simulink model "Z_3DCtrl_xiaodong"  (R2022a)
settings: Solver=ode1  StartTime=0.0  StopTime=Inf  FixedStep=0.001  RelTol=1e-3  EnableMultiTasking=on
PostLoadFcn:
  | , if any(exist('dsrtsu_mdlpostloadfcn', 'file') ~= 0), dsrtsu_mdlpostloadfcn('Execute', bdroot); end,
InitFcn:
  | , if any(exist('rtifpga_mdlclblib', 'file') ~= 0), rtifpga_mdlclblib('Init', bdroot); end,
  | [b,a] = butter(6,0.6)
undefined symbols (not defined in the file): a, b, DiscIntNeverNeededParam
libraries: simulink x3, rti2004lib x3, rtilibm x1
settings Model: DSRTSU_INTERNAL_RTI_VER=600  DSRTSU_INTERNAL_RTI_TYPE=rti1006  DSRTSU_INTERNAL_RTIFPGA=180  DSRTSU_INTERNAL_RTISTBM_VER=1.4.4  Creator=Administrator  LastModifiedBy=jnofech
settings SolverCC: AlgebraicLoopSolver=TrustRegion
settings DataIOCC: LimitDataPoints=on  SaveFormat=Array  SignalLoggingSaveFormat=ModelDataLogs  ReturnWorkspaceOutputs=off
settings OptimizationCC: BlockReduction=off  OptimizeBlockIOStorage=off  BufferReuse=off  ExpressionFolding=off  ExpressionDepthLimit=2147483647  LocalBlockOutputs=off  LifeSpan=inf
settings DebuggingCC: UnderspecifiedInitializationDetection=Classic  MergeDetectMultiDrivingBlocksExec=none  SolverPrmCheckMsg=warning  FcnCallInpInsideContextMsg=warning  UnconnectedInputMsg=warning  UnconnectedOutputMsg=warning  UnconnectedLineMsg=warning  StateNameClashWarn=warning  SFUnexpectedBacktrackingDiag=warning  SFNoUnconditionalDefaultTransitionDiag=warning  SFExecutionAtInitializationDiag=none  SFMachineParentedDataDiag=warning  ArithmeticOperatorsInVariantConditions=warning
settings HardwareCC: ProdBitPerPointer=32  ProdBitPerSizeT=32  ProdBitPerPtrDiffT=32  ProdLargestAtomicInteger=Integer  ProdWordSize=32  ProdHWDeviceType=Custom Processor->Custom  TargetIntDivRoundTo=Zero  TargetEndianess=LittleEndian  TargetHWDeviceType=Custom Processor->Custom
settings ModelReferenceCC: PropagateSignalLabelsOutOfModel=off
settings SFSimCC: SimUseLocalCustomCode=off  MATLABDynamicMemAlloc=off  CustomCodeUndefinedFunction=UseInterfaceOnly
settings RTWCC: Description=dSPACE DS1006 Hardware Platform  SystemTargetFile=rti1006.tlc  MakeCommand=make_rti  TemplateMakefile=rti1006.tmf  RTWUseLocalCustomCode=off
settings CodeAppCC: StateflowObjectComments=on
settings STFCustomTargetCC: ParMdlRefBuildCompliant=on  GRTInterface=off  SystemTargetFile=rti1006.tlc
settings GRTTargetCC: TargetLangStandard=C89/C90 (ANSI)  CompOptLevelCompliant=off  ConcurrentExecutionCompliant=off  CombineOutputUpdateFcns=off  MatFileLogging=off  CPPClassGenCompliant=off  UseToolchainInfoCompliant=off  ExtModeMexFile=noextcomm
settings ConfigComp: CovMetricSettings=dw  CovSaveCumulativeToWorkspaceVar=on  CovSaveSingleToWorkspaceVar=on

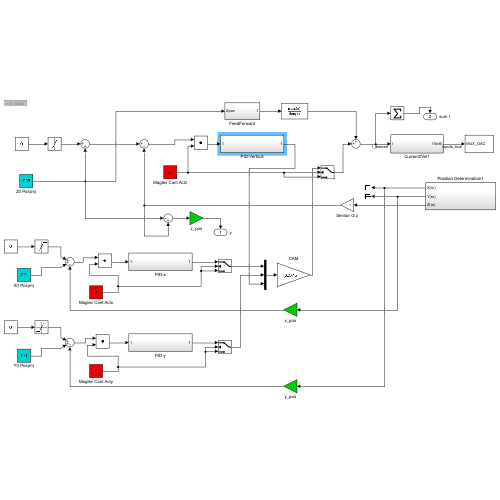
[thumbnail: Simulink's stored preview of the top-level diagram]
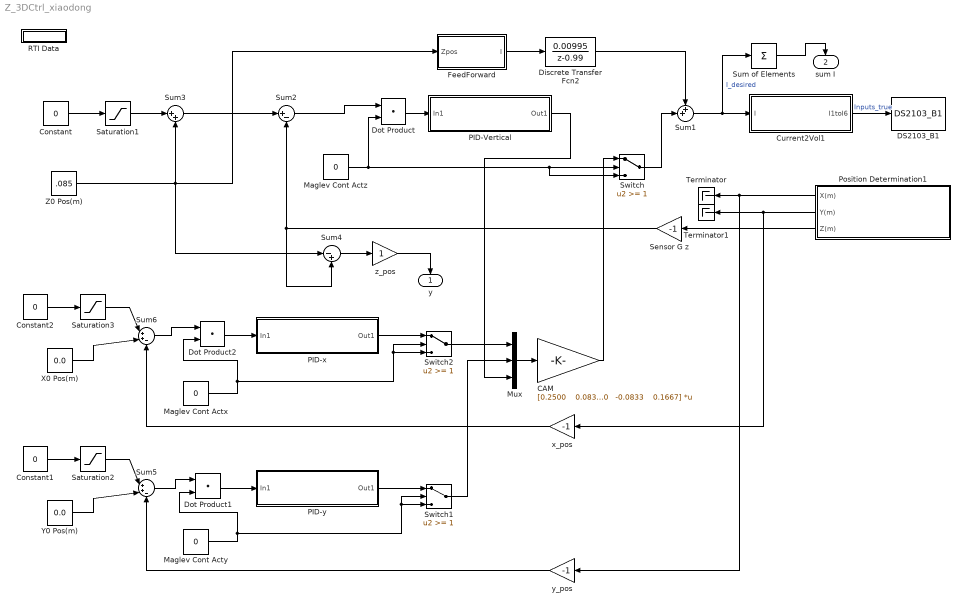
== system Z_3DCtrl_xiaodong ==
  CAM : Gain  Gain=|  Multiplication=Matrix(K*u)
      | [0.2500    0.0833    0.1667
      |          0    0.1667    0.1667
      |    -0.2500    0.0833    0.1667
      |    -0.2500   -0.0833    0.1667
      |          0   -0.1667    0.1667
      |     0.2500   -0.0833    0.1667]
  Constant : Constant  Value=0
  Constant1 : Constant  Value=0
  Constant2 : Constant  Value=0
  Current2Vol1 : Subsystem
  DS2103_B1 : rtilibm/DS2103/DS2103_B1  BoardNo=1  ChannelNos=[1 2 4 6 8 9 10 11 12 18 19 20]  Range=[10 10 10 10 10 10 10 10 10 10 10 10 10 10 10 10 10 10 10 10 10 10 10 10 10 10 10 10 10 10 10 10]  IOErrorMode=[1 1 1 1 1 1 1 1]  InitValue=[0 0 0 0 0 0 0 0 0 0 0 0 0 0 0 0 0 0 0 0 0 0 0 0 0 0 0 0 0 0 0 0]  TermMode=[0 0 0 0 0 0 0 1 1 1 1 1 1 1 1 1 1 1 1 1 1 1 1 1 1 1 1 1 1 1 1 1]  TermValue=[0 0 0 0 0 0 0 0 0 0 0 0 0 0 0 0 0 0 0 0 0 0 0 0 0 0 0 0 0 0 0 0]  DialogFcn=gui2103  UnitName={ 'DS2103_B' }  UnitValues={ 1 }  DSProperties=struct('RTI',struct('Version',uint32(1),'BlockType',struct('isSLSource',uint8(0),'isSLSink',uint8(1),'isHWSource',uint8(0),'isHWSink',uint8(1),'isSetup',uint8(0),'isInline',uint8(1),'isNonInline',uint8(0),'isInterrupt',uint8(0),'isChannelwise',uint8(0)),'IOBoardType','DS2103','UnitType','DAC','Identifier','DACMUX','DialogType','ML','BlockSet','NONE','SlaveProcessor','NONE'))
      settings: SourceProductName=dSPACE RTI1006
  Discrete Transfer Fcn2 : DiscreteTransferFcn  Numerator=[0.00995]  Denominator=[1 -0.99]
  Dot Product : DotProduct  OutDataTypeStr=Inherit: Inherit via internal rule
  Dot Product1 : DotProduct  OutDataTypeStr=Inherit: Inherit via internal rule
  Dot Product2 : DotProduct  OutDataTypeStr=Inherit: Inherit via internal rule
  FeedForward : Subsystem
  Maglev Cont Actx : Constant  Value=0
  Maglev Cont Acty : Constant  Value=0
  Maglev Cont Actz : Constant  Value=0
  Mux : Mux  Inputs=3
  PID-Vertical : Subsystem
  PID-x : Subsystem
  PID-y : Subsystem
  Position Determination1 : Subsystem
  RTI Data : Subsystem  Tag=struct('RTIDataServer',struct('RTIDataServerVs','2','RTIModelDescription','struct(''main'',''Z_3DCtrl_xiaodong'',''sub'','''',''isMp'',0)'))  LoadFcn="if exist('rtidc'), try,  rtidc('DataHostBlockClbLoad', gcbh); catch, disp(['Warning: ''LoadFcn'' for RTI Data block failed: ' lasterr]); end, end,"  mask(RTI_DATA_HOST){}
      mask help:
      | RTI Data Block.
      | This block is used by RTI to store internal model-dependent data.
      | Please keep this block on the root level of the model. Deleting this block will result in data loss.
      |
      | NEVER DELETE OR COPY THIS BLOCK!
      settings: CopyFcn="if exist('rtidc'), try,  rtidc('DataHostBlockClbCopy', gcbh); catch, disp(['Warning: ''CopyFcn'' for RTI Data block failed: ' lasterr]); end, end,"  DeleteFcn="if exist('rtidc'), try,  rtidc('DataHostBlockClbDelete', gcbh); catch, disp(['Warning: ''DeleteFcn'' for RTI Data block failed: ' lasterr]); end, end,"  ModelCloseFcn="if exist('rtidc'), try,  rtidc('DataHostBlockClbModelClose', gcbh); catch, disp(['Warning: ''ModelCloseFcn'' for RTI Data block failed: ' lasterr]); end, end,"  PreSaveFcn="if exist('rtidc'), try,  rtidc('DataHostBlockClbPreSave', gcbh); catch, disp(['Warning: ''PreSaveFcn'' for RTI Data block failed: ' lasterr]); end, end,"  PostSaveFcn="if exist('rtidc'), try,  rtidc('DataHostBlockClbPostSave', gcbh); catch, disp(['Warning: ''PostSaveFcn'' for RTI Data block failed: ' lasterr]); end, end,"  NameChangeFcn="if exist('rtidc'), try,  rtidc('DataHostBlockClbNameChange', gcbh); catch, disp(['Warning: ''NameChangeFcn'' for RTI Data block failed: ' lasterr]); end, end,"
      mask Help:
      | RTI Data Block.
      | This block is used by RTI to store internal model-dependent data.
      | Please keep this block on the root level of the model. Deleting this block will result in data loss.
      | 
      | NEVER DELETE OR COPY THIS BLOCK!
      mask Display:
      | text(0.5, 0.5, 'RTI Data', 'HorizontalAlignment', 'center');
      | plot([1 0]);
  Saturation1 : Saturate  UpperLimit=.015  LowerLimit=-.015
  Saturation2 : Saturate  UpperLimit=.01  LowerLimit=-.01
  Saturation3 : Saturate  UpperLimit=.01  LowerLimit=-.01
  Sensor G z : Gain  Gain=-1
  Sum of Elements : Sum  Inputs=+
  Sum1 : Sum  Inputs=++|
  Sum2 : Sum  Inputs=|+-
  Sum3 : Sum  Inputs=|++
  Sum4 : Sum  Inputs=|-+
  Sum5 : Sum  Inputs=|++-
  Sum6 : Sum  Inputs=|++-
  Switch : Switch  Threshold=1  SaturateOnIntegerOverflow=off  InputSameDT=off
  Switch1 : Switch  Threshold=1  SaturateOnIntegerOverflow=off  InputSameDT=off
  Switch2 : Switch  Threshold=1  SaturateOnIntegerOverflow=off  InputSameDT=off
  Terminator : Terminator
  Terminator1 : Terminator
  X0 Pos(m) : Constant  Value=0.0
  Y0 Pos(m) : Constant  Value=0.0
  Z0 Pos(m) : Constant  Value=.085
  x_pos : Gain  Gain=-1
  y_pos : Gain  Gain=-1
  z_pos : Gain
  y : Outport
  sum I : Outport  Port=2
  wires:
  Sum1/1 -> Sum of Elements/1, Current2Vol1/1(I)  "I_desired"
  Sum3/1 -> Sum2/1
  Position Determination1/3(Z(m)) -> Sensor G z/1
  Position Determination1/1(X(m)) -> Terminator/1, y_pos/1
  Position Determination1/2(Y(m)) -> Terminator1/1, x_pos/1
  Sensor G z/1 -> Sum2/2, Sum4/2
  FeedForward/1(I) -> Discrete Transfer Fcn2/1
  Constant/1 -> Saturation1/1
  Saturation1/1 -> Sum3/1
  Sum4/1 -> z_pos/1
  Maglev Cont Actz/1 -> Switch/2, Switch/3, Dot Product/2
  Switch/1 -> Sum1/2
  Dot Product/1 -> PID-Vertical/1(In1)
  Sum2/1 -> Dot Product/1
  Mux/1 -> CAM/1
  CAM/1 -> Switch/1
  PID-Vertical/1(Out1) -> Mux/3
  Constant1/1 -> Saturation2/1
  Saturation2/1 -> Sum5/1
  Discrete Transfer Fcn2/1 -> Sum1/1
  Sum of Elements/1 -> sum I/1
  Sum5/1 -> Dot Product1/1
  Dot Product1/1 -> PID-y/1(In1)
  Maglev Cont Acty/1 -> Dot Product1/2, Switch1/3, Switch1/2
  PID-y/1(Out1) -> Switch1/1
  Switch1/1 -> Mux/2
  Constant2/1 -> Saturation3/1
  Saturation3/1 -> Sum6/1
  Sum6/1 -> Dot Product2/1
  Dot Product2/1 -> PID-x/1(In1)
  Maglev Cont Actx/1 -> Switch2/2, Switch2/3, Dot Product2/2
  PID-x/1(Out1) -> Switch2/1
  Switch2/1 -> Mux/1
  X0 Pos(m)/1 -> Sum6/2
  Y0 Pos(m)/1 -> Sum5/2
  Z0 Pos(m)/1 -> Sum3/2, FeedForward/1(Zpos), Sum4/1
  x_pos/1 -> Sum6/3
  y_pos/1 -> Sum5/3
  z_pos/1 -> y/1
  Current2Vol1/1(I1toI6) -> DS2103_B1/1  "Inputs_true"

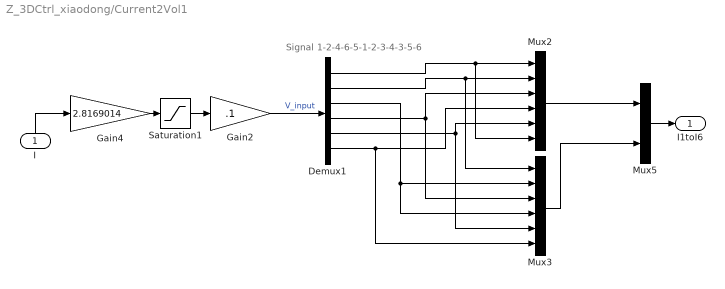
== system Z_3DCtrl_xiaodong/Current2Vol1 ==
  note: Signal 1-2-4-6-5-1-2-3-4-3-5-6
  I : Inport
  Demux1 : Demux  Outputs=6
  Gain2 : Gain  Gain=.1
  Gain4 : Gain  Gain=2.8169014
  Mux2 : Mux  Inputs=6
  Mux3 : Mux  Inputs=6
  Mux5 : Mux  Inputs=2
  Saturation1 : Saturate  UpperLimit=8.2  LowerLimit=0
  I1toI6 : Outport
  wires:
  Mux5/1 -> I1toI6/1
  I/1 -> Gain4/1
  Gain4/1 -> Saturation1/1
  Mux2/1 -> Mux5/1
  Saturation1/1 -> Gain2/1
  Gain2/1 -> Demux1/1  "V_input"
  Mux3/1 -> Mux5/2
  Demux1/1 -> Mux2/1, Mux2/6
  Demux1/2 -> Mux2/2, Mux3/1
  Demux1/4 -> Mux2/3, Mux3/3
  Demux1/6 -> Mux2/4, Mux3/6
  Demux1/5 -> Mux2/5, Mux3/5
  Demux1/3 -> Mux3/2, Mux3/4

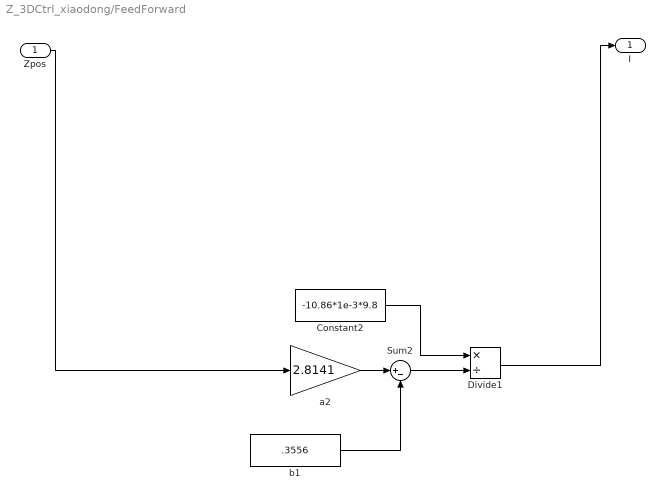
== system Z_3DCtrl_xiaodong/FeedForward ==
  Zpos : Inport
  Constant2 : Constant  Value=-10.86*1e-3*9.8
  Divide1 : Product  Inputs=*/
  Sum2 : Sum  Inputs=|+-
  a2 : Gain  Gain=2.8141
  b1 : Constant  Value=.3556
  I : Outport
  wires:
  a2/1 -> Sum2/1
  b1/1 -> Sum2/2
  Zpos/1 -> a2/1
  Constant2/1 -> Divide1/1
  Sum2/1 -> Divide1/2
  Divide1/1 -> I/1

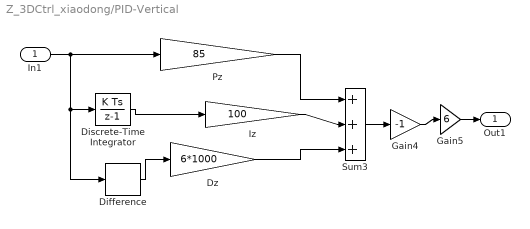
== system Z_3DCtrl_xiaodong/PID-Vertical ==
  In1 : Inport
  Difference : simulink/Discrete/Difference  ICPrevInput=0.0  OutMin=[]  OutMax=[]  OutDataType=sfix(16)  OutScaling=2^-10  DoSatur=off
  Discrete-Time Integrator : DiscreteIntegrator  SampleTime=-1  ICPrevOutput=DiscIntNeverNeededParam  ICPrevScaledInput=DiscIntNeverNeededParam
  Dz : Gain  Gain=6*1000
  Gain4 : Gain  Gain=-1
  Gain5 : Gain  Gain=6
  Iz : Gain  Gain=100
  Pz : Gain  Gain=85
  Sum3 : Sum  Inputs=|+++
  Out1 : Outport
  wires:
  Pz/1 -> Sum3/1
  Difference/1 -> Dz/1
  Iz/1 -> Sum3/2
  Dz/1 -> Sum3/3
  In1/1 -> Pz/1, Difference/1, Discrete-Time Integrator/1
  Sum3/1 -> Gain4/1
  Gain4/1 -> Gain5/1
  Gain5/1 -> Out1/1
  Discrete-Time Integrator/1 -> Iz/1

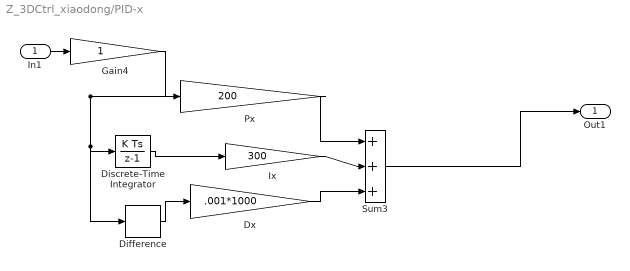
== system Z_3DCtrl_xiaodong/PID-x ==
  In1 : Inport
  Difference : simulink/Discrete/Difference  ICPrevInput=0.0  OutMin=[]  OutMax=[]  OutDataType=sfix(16)  OutScaling=2^-10  DoSatur=off
  Discrete-Time Integrator : DiscreteIntegrator  SampleTime=-1  ICPrevOutput=DiscIntNeverNeededParam  ICPrevScaledInput=DiscIntNeverNeededParam
  Dx : Gain  Gain=.001*1000
  Gain4 : Gain
  Ix : Gain  Gain=300
  Px : Gain  Gain=200
  Sum3 : Sum  Inputs=|+++
  Out1 : Outport
  wires:
  In1/1 -> Gain4/1
  Px/1 -> Sum3/1
  Difference/1 -> Dx/1
  Ix/1 -> Sum3/2
  Dx/1 -> Sum3/3
  Discrete-Time Integrator/1 -> Ix/1
  Gain4/1 -> Px/1, Difference/1, Discrete-Time Integrator/1
  Sum3/1 -> Out1/1

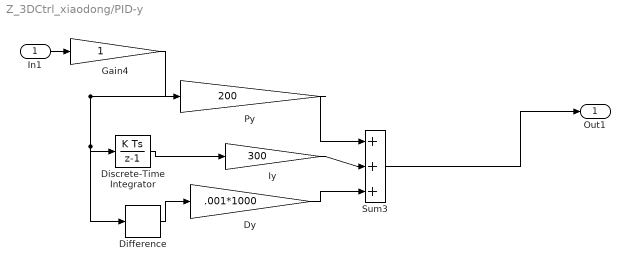
== system Z_3DCtrl_xiaodong/PID-y ==
  In1 : Inport
  Difference : simulink/Discrete/Difference  ICPrevInput=0.0  OutMin=[]  OutMax=[]  OutDataType=sfix(16)  OutScaling=2^-10  DoSatur=off
  Discrete-Time Integrator : DiscreteIntegrator  SampleTime=-1  ICPrevOutput=DiscIntNeverNeededParam  ICPrevScaledInput=DiscIntNeverNeededParam
  Dy : Gain  Gain=.001*1000
  Gain4 : Gain
  Iy : Gain  Gain=300
  Py : Gain  Gain=200
  Sum3 : Sum  Inputs=|+++
  Out1 : Outport
  wires:
  In1/1 -> Gain4/1
  Py/1 -> Sum3/1
  Difference/1 -> Dy/1
  Iy/1 -> Sum3/2
  Dy/1 -> Sum3/3
  Discrete-Time Integrator/1 -> Iy/1
  Gain4/1 -> Py/1, Difference/1, Discrete-Time Integrator/1
  Sum3/1 -> Out1/1

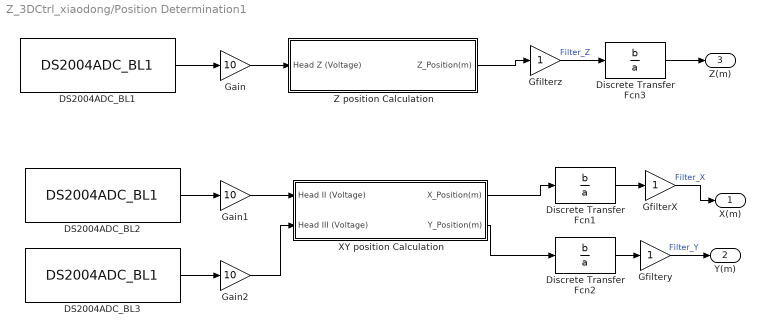
== system Z_3DCtrl_xiaodong/Position Determination1 ==
  DS2004ADC_BL1 : rti2004lib/DS2004ADC_BL1  DSProperties=struct('RTI',struct('Version',uint32(1),'BlockType',struct('isSLSource',uint8(1),'isSLSink',uint8(1),'isHWSource',uint8(0),'isHWSink',uint8(1),'isSetup',uint8(0),'isInline',uint8(1),'isNonInline',uint8(0),'isInterrupt',uint8(0),'isChannelwise',uint8(1)),'IOBoardType','DS2004','UnitType','ADC','Identifier','ADC','DialogType','ML','BlockSet','NONE','SlaveProcessor','NONE'))  RTIBlockInterface=struct('InputPortsActive',0,'InputPortsWidth',int32(1),'InputPortsDataType',{{'SS_BOOLEAN'}},'InputPortsName',{{'Continue'}},'OutputPortsActive',[1 0],'OutputPortsWidth',int32([1 1]),'OutputPortsDataType',{{'SS_DOUBLE','SS_UINT8'}},'OutputPortsName',{{'ADC','Status'}},'DialogFcn','rti2004adcgui','SampleTime',{{-1}},'InitLevel',3,'IconTransparency','on','BlockDisplay',{{['DS2004 ADC\nBoard: 1\nChannel: 1'],'center'}},'BlockName',struct('Token',{{'DS2004ADC_BL1'}}))  RTIBlockParameters=struct('ADCSWStartDisable',{{0,'OFF',[0 1]}},'BoardNo',{{1,'OFF',[1 16]}},'ChannelNo',{{1,'OFF',[1 16]}},'ConversionMode',{{1,'OFF',[1 2]}},'SampleMode',{{1,'OFF',[1 2]}},'TriggerSource',{{1,'OFF',[1 5]}},'EdgePolarity',{{1,'OFF',[1 2]}},'ConversionTriggerSource',{{2,'OFF',[1 6]}},'ConversionEdgePolarity',{{1,'OFF',[1 2]}},'ConversionPeriod',{{1e-6,'OFF',[]}},'ConversionPeriodCheck',{{0,'OFF',[]}},'BurstTriggerSource',{{1,'OFF',[1 6]}},'BurstEdgePolarity',{{1,'OFF',[1 2]}},'BurstSize',{{10,'OFF',[]}},'BurstSizeCheck',{{0,'OFF',[]}},'DataSetOffset',{{0,'OFF',[]}},'DataSetOffsetCheck',{{0,'OFF',[]}},'DataSetLength',{{1,'OFF',[]}},'DataSetLengthCheck',{{0,'OFF',[]}},'ReadMode',{{1,'OFF',[1 2]}},'SampleTime',{{-1,'OFF',[-1 inf]}},'SampleTimeCheck',{{1,'OFF',[]}},'InputVoltageRange',{{2,'OFF',[1 2]}},'StatusPortEnable',{{0,'OFF',[0 1]}},'TLCFileName',{{'rti2004adc','OFF',[]}})  RTISFcnParameters=struct('ADCSWStartDisable','int32','BoardNo','int32','ChannelNo','int32','ConversionMode','int32','SampleMode','int32','TriggerSource','int32','EdgePolarity','int32','ConversionTriggerSource','int32','ConversionEdgePolarity','int32','ConversionPeriod','double','BurstTriggerSource','int32','BurstEdgePolarity','int32','BurstSize','int32','DataSetOffset','int32','DataSetLength','int32','ReadMode','int32','SampleTime','double','InputVoltageRange','int32','StatusPortEnable','int32','TLCFileName','char')  RTIBlockParaDefault=struct('ADCSWStartDisable',0,'BoardNo',1,'ChannelNo',1,'ConversionMode',1,'SampleMode',1,'TriggerSource',1,'EdgePolarity',1,'ConversionTriggerSource',2,'ConversionEdgePolarity',1,'ConversionPeriod',1e-6,'ConversionPeriodCheck',0,'BurstTriggerSource',1,'BurstEdgePolarity',1,'BurstSize',10,'BurstSizeCheck',0,'DataSetOffset',0,'DataSetOffsetCheck',0,'DataSetLength',1,'DataSetLengthCheck',0,'ReadMode',1,'SampleTime',-1,'SampleTimeCheck',1,'InputVoltageRange',2,'StatusPortEnable',0,'TLCFileName','rti2004adc')
  DS2004ADC_BL2 : rti2004lib/DS2004ADC_BL1  DSProperties=struct('RTI',struct('Version',uint32(1),'BlockType',struct('isSLSource',uint8(1),'isSLSink',uint8(1),'isHWSource',uint8(0),'isHWSink',uint8(1),'isSetup',uint8(0),'isInline',uint8(1),'isNonInline',uint8(0),'isInterrupt',uint8(0),'isChannelwise',uint8(1)),'IOBoardType','DS2004','UnitType','ADC','Identifier','ADC','DialogType','ML','BlockSet','NONE','SlaveProcessor','NONE'))  RTIBlockInterface=struct('InputPortsActive',0,'InputPortsWidth',int32(1),'InputPortsDataType',{{'SS_BOOLEAN'}},'InputPortsName',{{'Continue'}},'OutputPortsActive',[1 0],'OutputPortsWidth',int32([1 1]),'OutputPortsDataType',{{'SS_DOUBLE','SS_UINT8'}},'OutputPortsName',{{'ADC','Status'}},'DialogFcn','rti2004adcgui','SampleTime',{{-1}},'InitLevel',3,'IconTransparency','on','BlockDisplay',{{['DS2004 ADC\nBoard: 1\nChannel: 2'],'center'}},'BlockName',struct('Token',{{'DS2004ADC_BL1'}}))  RTIBlockParameters=struct('ADCSWStartDisable',{{0,'OFF',[0 1]}},'BoardNo',{{1,'OFF',[1 16]}},'ChannelNo',{{2,'OFF',[1 16]}},'ConversionMode',{{1,'OFF',[1 2]}},'SampleMode',{{1,'OFF',[1 2]}},'TriggerSource',{{1,'OFF',[1 5]}},'EdgePolarity',{{1,'OFF',[1 2]}},'ConversionTriggerSource',{{2,'OFF',[1 6]}},'ConversionEdgePolarity',{{1,'OFF',[1 2]}},'ConversionPeriod',{{'1e-006','OFF',[]}},'ConversionPeriodCheck',{{0,'OFF',[]}},'BurstTriggerSource',{{1,'OFF',[1 6]}},'BurstEdgePolarity',{{1,'OFF',[1 2]}},'BurstSize',{{'10','OFF',[]}},'BurstSizeCheck',{{0,'OFF',[]}},'DataSetOffset',{{'0','OFF',[]}},'DataSetOffsetCheck',{{0,'OFF',[]}},'DataSetLength',{{'1','OFF',[]}},'DataSetLengthCheck',{{0,'OFF',[]}},'ReadMode',{{1,'OFF',[1 2]}},'SampleTime',{{'-1','OFF',[-1 inf]}},'SampleTimeCheck',{{1,'OFF',[]}},'InputVoltageRange',{{2,'OFF',[1 2]}},'StatusPortEnable',{{0,'OFF',[0 1]}},'TLCFileName',{{'rti2004adc','OFF',[]}})  RTISFcnParameters=struct('ADCSWStartDisable','int32','BoardNo','int32','ChannelNo','int32','ConversionMode','int32','SampleMode','int32','TriggerSource','int32','EdgePolarity','int32','ConversionTriggerSource','int32','ConversionEdgePolarity','int32','ConversionPeriod','double','BurstTriggerSource','int32','BurstEdgePolarity','int32','BurstSize','int32','DataSetOffset','int32','DataSetLength','int32','ReadMode','int32','SampleTime','double','InputVoltageRange','int32','StatusPortEnable','int32','TLCFileName','char')  RTIBlockParaDefault=struct('ADCSWStartDisable',0,'BoardNo',1,'ChannelNo',1,'ConversionMode',1,'SampleMode',1,'TriggerSource',1,'EdgePolarity',1,'ConversionTriggerSource',2,'ConversionEdgePolarity',1,'ConversionPeriod',1e-6,'ConversionPeriodCheck',0,'BurstTriggerSource',1,'BurstEdgePolarity',1,'BurstSize',10,'BurstSizeCheck',0,'DataSetOffset',0,'DataSetOffsetCheck',0,'DataSetLength',1,'DataSetLengthCheck',0,'ReadMode',1,'SampleTime',-1,'SampleTimeCheck',1,'InputVoltageRange',2,'StatusPortEnable',0,'TLCFileName','rti2004adc')
  DS2004ADC_BL3 : rti2004lib/DS2004ADC_BL1  DSProperties=struct('RTI',struct('Version',uint32(1),'BlockType',struct('isSLSource',uint8(1),'isSLSink',uint8(1),'isHWSource',uint8(0),'isHWSink',uint8(1),'isSetup',uint8(0),'isInline',uint8(1),'isNonInline',uint8(0),'isInterrupt',uint8(0),'isChannelwise',uint8(1)),'IOBoardType','DS2004','UnitType','ADC','Identifier','ADC','DialogType','ML','BlockSet','NONE','SlaveProcessor','NONE'))  RTIBlockInterface=struct('InputPortsActive',0,'InputPortsWidth',int32(1),'InputPortsDataType',{{'SS_BOOLEAN'}},'InputPortsName',{{'Continue'}},'OutputPortsActive',[1 0],'OutputPortsWidth',int32([1 1]),'OutputPortsDataType',{{'SS_DOUBLE','SS_UINT8'}},'OutputPortsName',{{'ADC','Status'}},'DialogFcn','rti2004adcgui','SampleTime',{{-1}},'InitLevel',3,'IconTransparency','on','BlockDisplay',{{['DS2004 ADC\nBoard: 1\nChannel: 3'],'center'}},'BlockName',struct('Token',{{'DS2004ADC_BL1'}}))  RTIBlockParameters=struct('ADCSWStartDisable',{{0,'OFF',[0 1]}},'BoardNo',{{1,'OFF',[1 16]}},'ChannelNo',{{3,'OFF',[1 16]}},'ConversionMode',{{1,'OFF',[1 2]}},'SampleMode',{{1,'OFF',[1 2]}},'TriggerSource',{{1,'OFF',[1 5]}},'EdgePolarity',{{1,'OFF',[1 2]}},'ConversionTriggerSource',{{2,'OFF',[1 6]}},'ConversionEdgePolarity',{{1,'OFF',[1 2]}},'ConversionPeriod',{{'1e-006','OFF',[]}},'ConversionPeriodCheck',{{0,'OFF',[]}},'BurstTriggerSource',{{1,'OFF',[1 6]}},'BurstEdgePolarity',{{1,'OFF',[1 2]}},'BurstSize',{{'10','OFF',[]}},'BurstSizeCheck',{{0,'OFF',[]}},'DataSetOffset',{{'0','OFF',[]}},'DataSetOffsetCheck',{{0,'OFF',[]}},'DataSetLength',{{'1','OFF',[]}},'DataSetLengthCheck',{{0,'OFF',[]}},'ReadMode',{{1,'OFF',[1 2]}},'SampleTime',{{'-1','OFF',[-1 inf]}},'SampleTimeCheck',{{1,'OFF',[]}},'InputVoltageRange',{{2,'OFF',[1 2]}},'StatusPortEnable',{{0,'OFF',[0 1]}},'TLCFileName',{{'rti2004adc','OFF',[]}})  RTISFcnParameters=struct('ADCSWStartDisable','int32','BoardNo','int32','ChannelNo','int32','ConversionMode','int32','SampleMode','int32','TriggerSource','int32','EdgePolarity','int32','ConversionTriggerSource','int32','ConversionEdgePolarity','int32','ConversionPeriod','double','BurstTriggerSource','int32','BurstEdgePolarity','int32','BurstSize','int32','DataSetOffset','int32','DataSetLength','int32','ReadMode','int32','SampleTime','double','InputVoltageRange','int32','StatusPortEnable','int32','TLCFileName','char')  RTIBlockParaDefault=struct('ADCSWStartDisable',0,'BoardNo',1,'ChannelNo',1,'ConversionMode',1,'SampleMode',1,'TriggerSource',1,'EdgePolarity',1,'ConversionTriggerSource',2,'ConversionEdgePolarity',1,'ConversionPeriod',1e-6,'ConversionPeriodCheck',0,'BurstTriggerSource',1,'BurstEdgePolarity',1,'BurstSize',10,'BurstSizeCheck',0,'DataSetOffset',0,'DataSetOffsetCheck',0,'DataSetLength',1,'DataSetLengthCheck',0,'ReadMode',1,'SampleTime',-1,'SampleTimeCheck',1,'InputVoltageRange',2,'StatusPortEnable',0,'TLCFileName','rti2004adc')
  Discrete Transfer Fcn1 : DiscreteTransferFcn  Numerator=b  Denominator=a
  Discrete Transfer Fcn2 : DiscreteTransferFcn  Numerator=b  Denominator=a
  Discrete Transfer Fcn3 : DiscreteTransferFcn  Numerator=b  Denominator=a
  Gain : Gain  Gain=10
  Gain1 : Gain  Gain=10
  Gain2 : Gain  Gain=10
  GfilterX : Gain
  Gfiltery : Gain
  Gfilterz : Gain
  XY position Calculation : Subsystem
  Z position Calculation : Subsystem
  X(m) : Outport
  Y(m) : Outport  Port=2
  Z(m) : Outport  Port=3
  wires:
  Discrete Transfer Fcn2/1 -> Gfiltery/1
  Discrete Transfer Fcn1/1 -> GfilterX/1
  Gfilterz/1 -> Discrete Transfer Fcn3/1  "Filter_Z"
  GfilterX/1 -> X(m)/1  "Filter_X"
  Gfiltery/1 -> Y(m)/1  "Filter_Y"
  XY position Calculation/2(Y_Position(m)) -> Discrete Transfer Fcn2/1
  XY position Calculation/1(X_Position(m)) -> Discrete Transfer Fcn1/1
  Gain2/1 -> XY position Calculation/2(Head III (Voltage))
  Gain1/1 -> XY position Calculation/1(Head II (Voltage))
  DS2004ADC_BL3/1 -> Gain2/1
  DS2004ADC_BL2/1 -> Gain1/1
  Z position Calculation/1(Z_Position(m)) -> Gfilterz/1
  Gain/1 -> Z position Calculation/1(Head Z (Voltage))
  DS2004ADC_BL1/1 -> Gain/1
  Discrete Transfer Fcn3/1 -> Z(m)/1

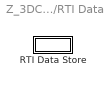
== system Z_3DCtrl_xiaodong/RTI Data ==
  RTI Data Store : Subsystem  Tag="struct('private',struct('version',struct('dsVer',uint32(2),'dsVerCreation',uint32(2),'RTI',struct('ver','6.2','type','RTI1006')),'access',struct('type','Model','isPerm',1,'created',['29-Jul-2010 10:53:51'],'modified',['25-Nov-2022 19:28:10'],'location','')),'public',struct('main',struct('data',[]),'sub',struct('name',{{'Z_3DCtrl_xiaodong'}},'data',{{struct('TH',struct('thTaskInfo',struct('taskType',{'TIMER','HWINT','TMRINT','SWINT','GLINT'},'tasksNumOf',{1,0,0,0,0},'srcIds',{{'TIMERA'},{},{},{},{}},'taskNames',{{['Timer Task 1']},{},{},{},{}})),'th_tc',struct('dataType','TASK','taskGroupId','','taskGroupList',{{}},'taskSchedulingPolicy','FCFS','taskType','TIMER','blkh',-1,'srcId','TIMERA','srcSgnName',['Timer A interrupt'],'srcCpuName','','taskName',['Timer Task 1  [0.001] s'],'taskNameDisplayExt','','smplTime',0.001,'smplTimeOffs',0,'hasFixedPriority',0,'priority',1,'hasFixedOvc',0,'ovcType',1,'ovcMax',1),'tc_th',struct('dataType','TASK','taskGroupId','','taskGroupList',{{}},'taskSchedulingPolicy','FCFS','taskType','TIMER','blkh',-1,'srcId','TIMERA','srcSgnName',['Timer A interrupt'],'srcCpuName','','taskName',['Timer Task 1  [0.001] s'],'taskNameDisplayExt','','smplTime',0.001,'smplTimeOffs',0,'hasFixedPriority',0,'priority',1,'hasFixedOvc',0,'ovcType',1,'ovcMax',1))}})))"  mask(RTI_DATA_STORE){}
      mask help:
      | RTI Data Store Block. This block is used by RTI to store internal model dependent data. Deleting this block will result in data loss.
      |
      | NEVER DELETE, COPY, OR MODIFY THIS BLOCK!
      mask Help:
      | RTI Data Store Block. This block is used by RTI to store internal model dependent data. Deleting this block will result in data loss.
      | 
      | NEVER DELETE, COPY, OR MODIFY THIS BLOCK!
      mask Display: text(0.5, 0.5, ' ', 'HorizontalAlignment', 'center');

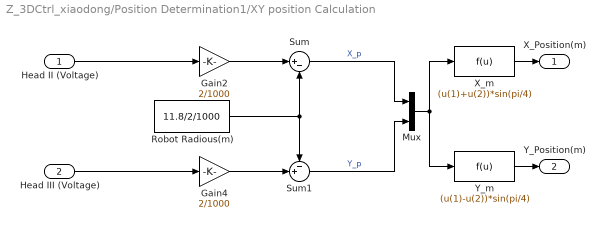
== system Z_3DCtrl_xiaodong/Position Determination1/XY position Calculation ==
  Head II (Voltage) : Inport
  Head III (Voltage) : Inport  Port=2
  Gain2 : Gain  Gain=2/1000
  Gain4 : Gain  Gain=2/1000
  Mux : Mux  Inputs=2
  Robot Radious(m) : Constant  Value=11.8/2/1000
  Sum : Sum  Inputs=|+-
  Sum1 : Sum  Inputs=-+|
  X_m : Fcn  Expr=(u(1)+u(2))*sin(pi/4)
  Y_m : Fcn  Expr=(u(1)-u(2))*sin(pi/4)
  X_Position(m) : Outport
  Y_Position(m) : Outport  Port=2
  wires:
  Head III (Voltage)/1 -> Gain4/1
  Y_m/1 -> Y_Position(m)/1
  X_m/1 -> X_Position(m)/1
  Head II (Voltage)/1 -> Gain2/1
  Mux/1 -> Y_m/1, X_m/1
  Sum1/1 -> Mux/2  "Y_p"
  Gain4/1 -> Sum1/2
  Sum/1 -> Mux/1  "X_p"
  Robot Radious(m)/1 -> Sum1/1, Sum/2
  Gain2/1 -> Sum/1

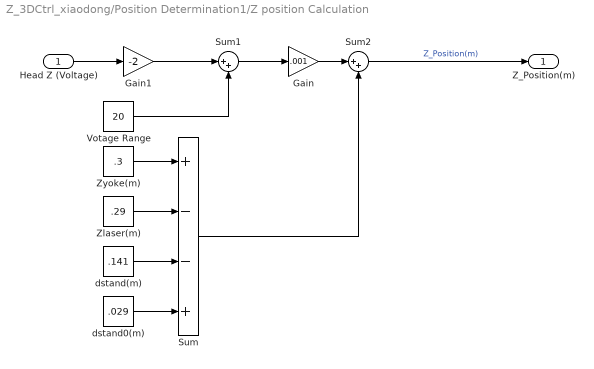
== system Z_3DCtrl_xiaodong/Position Determination1/Z position Calculation ==
  Head Z (Voltage) : Inport
  Gain : Gain  Gain=.001
  Gain1 : Gain  Gain=-2
  Sum : Sum  Inputs=+--+
  Sum1 : Sum  Inputs=|++
  Sum2 : Sum  Inputs=|++
  Votage Range : Constant  Value=20
  Zlaser(m) : Constant  Value=.29
  Zyoke(m) : Constant  Value=.3
  dstand(m) : Constant  Value=.141
  dstand0(m) : Constant  Value=.029
  Z_Position(m) : Outport
  wires:
  Sum2/1 -> Z_Position(m)/1  "Z_Position(m)"
  Head Z (Voltage)/1 -> Gain1/1
  Sum/1 -> Sum2/2
  Gain/1 -> Sum2/1
  Sum1/1 -> Gain/1
  Votage Range/1 -> Sum1/2
  Gain1/1 -> Sum1/1
  Zlaser(m)/1 -> Sum/2
  Zyoke(m)/1 -> Sum/1
  dstand(m)/1 -> Sum/3
  dstand0(m)/1 -> Sum/4

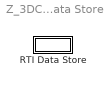
== system Z_3DCtrl_xiaodong/RTI Data/RTI Data Store ==
  RTI Data Store : Subsystem  mask(RTI_DATA_STORE){}
      mask help:
      | RTI Data Store Block. This block is used by RTI to store internal model dependent data. Deleting this block will result in data loss.
      |
      | NEVER DELETE, COPY, OR MODIFY THIS BLOCK!
      mask Help:
      | RTI Data Store Block. This block is used by RTI to store internal model dependent data. Deleting this block will result in data loss.
      | 
      | NEVER DELETE, COPY, OR MODIFY THIS BLOCK!
      mask Display: text(0.5, 0.5, ' ', 'HorizontalAlignment', 'center');

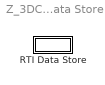
== system Z_3DCtrl_xiaodong/RTI Data/RTI Data Store/RTI Data Store ==
  RTI Data Store : Subsystem  mask(RTI_DATA_STORE){}
      mask help:
      | RTI Data Store Block. This block is used by RTI to store internal model dependent data. Deleting this block will result in data loss.
      |
      | NEVER DELETE, COPY, OR MODIFY THIS BLOCK!
      mask Help:
      | RTI Data Store Block. This block is used by RTI to store internal model dependent data. Deleting this block will result in data loss.
      | 
      | NEVER DELETE, COPY, OR MODIFY THIS BLOCK!
      mask Display: text(0.5, 0.5, ' ', 'HorizontalAlignment', 'center');

== system Z_3DCtrl_xiaodong/RTI Data/RTI Data Store/RTI Data Store/RTI Data Store ==
  RTI Data Store : Subsystem  mask(RTI_DATA_STORE){}
      mask help:
      | RTI Data Store Block. This block is used by RTI to store internal model dependent data. Deleting this block will result in data loss.
      |
      | NEVER DELETE, COPY, OR MODIFY THIS BLOCK!
      mask Help:
      | RTI Data Store Block. This block is used by RTI to store internal model dependent data. Deleting this block will result in data loss.
      | 
      | NEVER DELETE, COPY, OR MODIFY THIS BLOCK!
      mask Display: text(0.5, 0.5, ' ', 'HorizontalAlignment', 'center');

== system Z_3DCtrl_xiaodong/RTI Data/RTI Data Store/RTI Data Store/RTI Data Store/RTI Data Store ==
